simulink model "TORANonlinear"  (R2021a)
settings: Solver=VariableStepAuto  StartTime=0.0  StopTime=10.0  RelTol=1e-3
values from neighbouring files (symbols this model uses):
  A = [ 0 1      0 0 ... (first row only)    [epsysdyn.m]    (also in main_n10454012.m)
  B = [     0 ... (first row only)    [epsysdyn.m]    (also in main_n10454012.m)
  C = [ 0 0 0 0 ... (first row only)    [epsysdyn.m]    (also in kalmanfilter.m = [1 0 0 0]; main.m = [ 1 0 0 0; main_n10454012.m)
  controller_enabled = 1    [main.m]    (also in main_ClqrOkalmanI20deg0_1m.m; main_ClqrOoffI20deg0_1m.m; main_n10454012.m; maindefault.m)
  D = zeros(size(C, 1), size(B, 2))    [epsysdyn.m]    (also in main.m; main_n10454012.m)
  J = 0.0002175    [initialise.m]    (also in main_n10454012.m)
  K = place(A, B, [l1, l2, l3, l4])    [kSearch.m]    (also in main.m = Klqr; main_ClqrOkalmanI20deg0_1m.m = Klqr; main_ClqrOoffI20deg0_1m.m = Klqr; main_n10454012.m = Klqr)
  k = 186.3    [initialise.m]    (also in main_n10454012.m)
  L = 1    [initialise.m]    (also in main.m = Lnormal; main_ClqrOkalmanI20deg0_1m.m = Lkalman; main_ClqrOoffI20deg0_1m.m = Lkalman; main_n10454012.m = Lnormal)
  l = 0.2    [Cart_Pendulum_Animation.m]    (also in main_n10454012.m = 1)
  M = 1.3608    [initialise.m]    (also in main_n10454012.m)
  m = 0.096    [initialise.m]    (also in main_n10454012.m)
  R = diag([0.01*1 0.01*1])    [main.m]
  use_state_estimates = 1    [main.m]    (also in main_ClqrOkalmanI20deg0_1m.m; main_ClqrOoffI20deg0_1m.m = 0; main_n10454012.m; maindefault.m)
  x0 = [ 100*pi/180; 0; 0; 0 ]    [epsysdyn.m]    (also in main_n10454012.m = [ wrapTo180(20)*pi/180; 0; 0.1; 0 ])
  x_bar = xb_bar    [epsysdyn.m]    (also in main_n10454012.m)
  x_bar_obs = [x_bar(1); x_bar(3)]    [main.m]    (also in main_ClqrOkalmanI20deg0_1m.m; main_ClqrOoffI20deg0_1m.m; main_n10454012.m; maindefault.m)
undefined symbols (not defined in the file or in its folder): Continuous, Time
libraries: ctrlSharedLib x1
settings Model: Creator=chilla  LastModifiedBy=chilla
settings SolverCC: AlgebraicLoopSolver=TrustRegion
settings DebuggingCC: SFMachineParentedDataDiag=warning

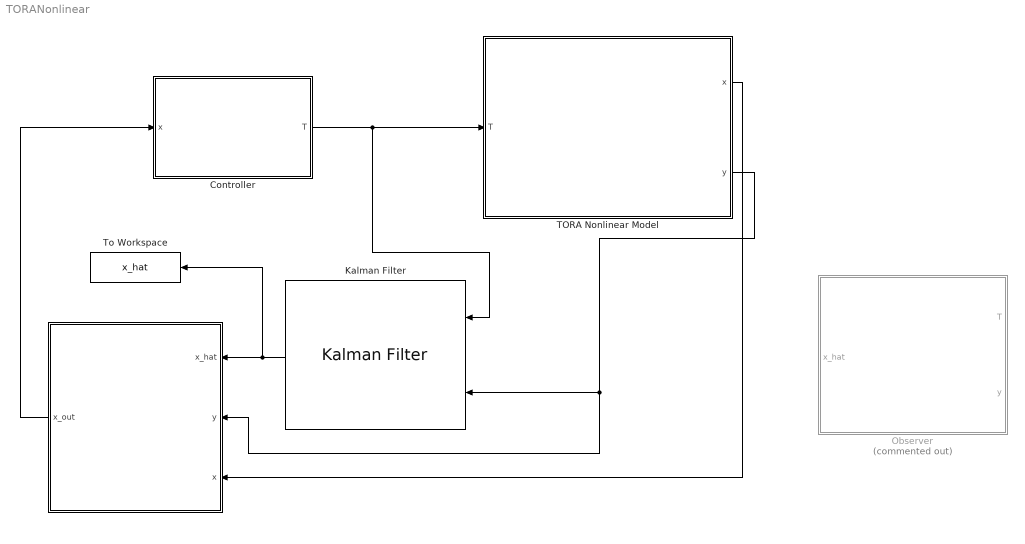
== system TORANonlinear ==
  " " : Subsystem
  Controller : Subsystem
  Kalman Filter : ctrlSharedLib/Kalman Filter  TimeDomain=Continuous-Time  UseCurrentEstimator=on  ModelSource=Individual A, B, C, D matrices  ModelSourceVariable=ss(0.95,1,1,0,1)  A=A  B=B  C=C  D=D  NumberOfStates=1  NumberOfInputs=1  NumberOfOutputs=1  InitialEstimateSource=Dialog  X0=0  P0=10  UseK=off  UseGH=off  NumberOfProcessNoiseInputs=1  G=1  TimeInvariantG=on  H=0  TimeInvariantH=on  Q=Q  TimeInvariantQ=on  R=R  TimeInvariantR=on  N=0  TimeInvariantN=on  AddInputPort=on  AddEnablePort=off  OutputEstimatedY=off  OutputP=off  Ts=-1
  Observer : Subsystem  Commented=on
  TORA Nonlinear Model : Subsystem
      mask Display: image('/Users/chilla/Downloads/TORA.png'); % Use "Edit Image" on toolstrip to change.
  To Workspace : ToWorkspace  VariableName=x_hat  SampleTime=-1
  wires:
  Controller/1(T) -> Kalman Filter/1, TORA Nonlinear Model/1(T)
  TORA Nonlinear Model/2(y) -> Kalman Filter/2, " "/2(y)
  TORA Nonlinear Model/1(x) -> " "/3(x)
  " "/1(x_out) -> Controller/1(x)
  Kalman Filter/1 -> To Workspace/1, " "/1(x_hat)

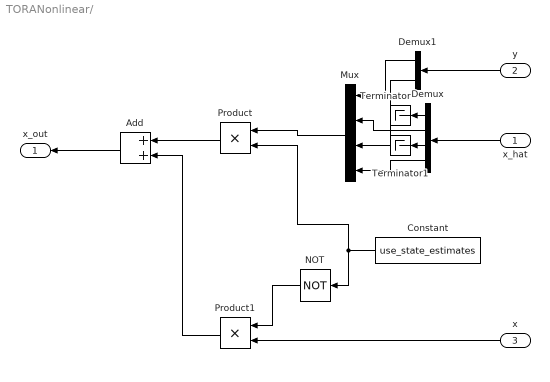
== system TORANonlinear/  ==
  x_hat : Inport
  y : Inport  Port=2
  x : Inport  Port=3
  Add : Sum
  Constant : Constant  Value=use_state_estimates
  Demux : Demux
  Demux1 : Demux  Outputs=2
  Mux : Mux
  NOT : Logic  Operator=NOT  IconShape=distinctive  AllPortsSameDT=off  OutDataTypeStr=boolean
  Product : Product
  Product1 : Product
  Terminator : Terminator
  Terminator1 : Terminator
  x_out : Outport
  wires:
  x_hat/1 -> Demux/1
  Mux/1 -> Product/1
  Constant/1 -> Product/2, NOT/1
  x/1 -> Product1/2
  NOT/1 -> Product1/1
  Add/1 -> x_out/1
  Product/1 -> Add/1
  Product1/1 -> Add/2
  Demux/1 -> Terminator/1
  Demux/3 -> Terminator1/1
  y/1 -> Demux1/1
  Demux/2 -> Mux/2
  Demux/4 -> Mux/4
  Demux1/1 -> Mux/1
  Demux1/2 -> Mux/3

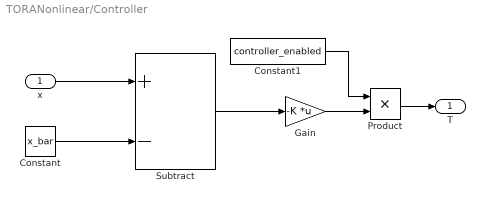
== system TORANonlinear/Controller ==
  x : Inport
  Constant : Constant  Value=x_bar
  Constant1 : Constant  Value=controller_enabled
  Gain : Gain  Gain=-K  Multiplication=Matrix(K*u)
  Product : Product
  Subtract : Sum  Inputs=+-
  T : Outport
  wires:
  Constant/1 -> Subtract/2
  Subtract/1 -> Gain/1
  x/1 -> Subtract/1
  Product/1 -> T/1
  Gain/1 -> Product/2
  Constant1/1 -> Product/1

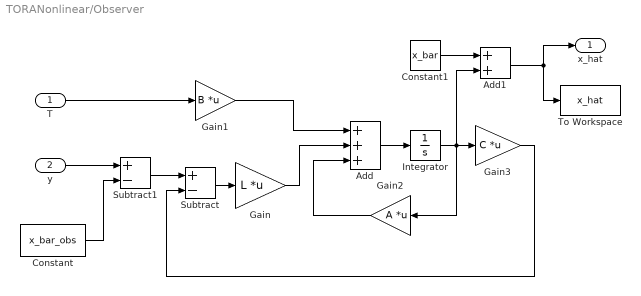
== system TORANonlinear/Observer ==
  T : Inport
  y : Inport  Port=2
  Add : Sum  Inputs=+++
  Add1 : Sum
  Constant : Constant  Value=x_bar_obs
  Constant1 : Constant  Value=x_bar
  Gain : Gain  Gain=L  Multiplication=Matrix(K*u)
  Gain1 : Gain  Gain=B  Multiplication=Matrix(K*u)
  Gain2 : Gain  Gain=A  Multiplication=Matrix(K*u)
  Gain3 : Gain  Gain=C  Multiplication=Matrix(K*u)
  Integrator : Integrator
  Subtract : Sum  Inputs=+-
  Subtract1 : Sum  Inputs=+-
  To Workspace : ToWorkspace  VariableName=x_hat  SampleTime=-1
  x_hat : Outport  VectorParamsAs1DForOutWhenUnconnected=off
  wires:
  Subtract/1 -> Gain/1
  T/1 -> Gain1/1
  Gain1/1 -> Add/1
  Gain/1 -> Add/2
  Add/1 -> Integrator/1
  Gain2/1 -> Add/3
  Gain3/1 -> Subtract/2
  y/1 -> Subtract1/1
  Subtract1/1 -> Subtract/1
  Constant/1 -> Subtract1/2
  Integrator/1 -> Add1/2, Gain2/1, Gain3/1
  Constant1/1 -> Add1/1
  Add1/1 -> To Workspace/1, x_hat/1

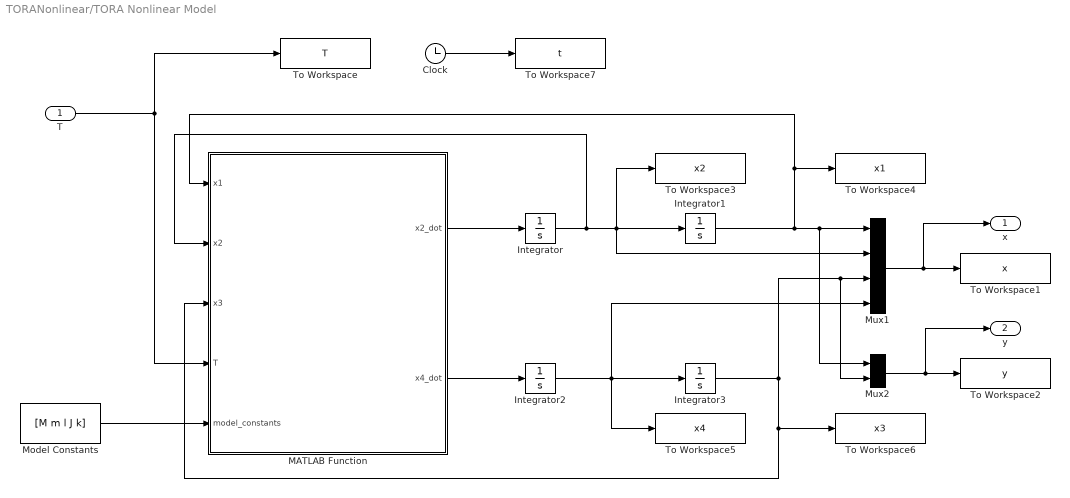
== system TORANonlinear/TORA Nonlinear Model ==
  T : Inport
  Clock : Clock
  Integrator : Integrator  InitialCondition=x0(2)
  Integrator1 : Integrator  InitialCondition=x0(1)
  Integrator2 : Integrator  InitialCondition=x0(4)
  Integrator3 : Integrator  InitialCondition=x0(3)
  MATLAB Function : MATLAB Function  TreatAsAtomicUnit=on
  Model Constants : Constant  Value=[M m l J k]
  Mux1 : Mux
  Mux2 : Mux  Inputs=2
  To Workspace : ToWorkspace  VariableName=T  SampleTime=-1
  To Workspace1 : ToWorkspace  VariableName=x  SampleTime=-1
  To Workspace2 : ToWorkspace  VariableName=y  SampleTime=-1
  To Workspace3 : ToWorkspace  VariableName=x2  SampleTime=-1
  To Workspace4 : ToWorkspace  VariableName=x1  SampleTime=-1
  To Workspace5 : ToWorkspace  VariableName=x4  SampleTime=-1
  To Workspace6 : ToWorkspace  VariableName=x3  SampleTime=-1
  To Workspace7 : ToWorkspace  VariableName=t  SampleTime=-1
  x : Outport
  y : Outport  Port=2
  wires:
  T/1 -> MATLAB Function/4(T), To Workspace/1
  Integrator/1 -> MATLAB Function/2(x2), To Workspace3/1, Integrator1/1, Mux1/2
  Integrator2/1 -> Integrator3/1, To Workspace5/1, Mux1/4
  Integrator3/1 -> Mux2/2, Mux1/3, MATLAB Function/3(x3), To Workspace6/1
  Mux2/1 -> y/1, To Workspace2/1
  Clock/1 -> To Workspace7/1
  MATLAB Function/1(x2_dot) -> Integrator/1
  Mux1/1 -> To Workspace1/1, x/1
  MATLAB Function/2(x4_dot) -> Integrator2/1
  Integrator1/1 -> MATLAB Function/1(x1), To Workspace4/1, Mux1/1, Mux2/1
  Model Constants/1 -> MATLAB Function/5(model_constants)

== matlab function TORANonlinear/TORA Nonlinear Model/MATLAB Function ==
  data: x1 input; x2_dot output; x2 input; x3 input; T input; x4_dot output; model_constants input
function [x2_dot, x4_dot] = NonLinearEquations(x1, x2, x3, T, model_constants)

% model constants
M = model_constants(1);
m = model_constants(2);
l = model_constants(3);
J = model_constants(4);
k = model_constants(5);

delTheta = (J + m*l^2)*(m + M) - m^2*l^2 * cos(x1)^2;
mid = (m*l*x2^2 * sin(x1) - k*x3);

x2_dot = ((m + M)*T  - m*l * cos(x1) * mid) / delTheta;
x4_dot = (-m*l*T * cos(x1) + (J + m*l^2) * mid) / delTheta;
